simulink model "sf_slswitch_nk"  (R2020a)
settings: Solver=FixedStepAuto  StartTime=0.0  StopTime=options.T_train  FixedStep=options.dt  MaxStep=.2  RelTol=1e-3
model workspace (MAT data in the model file):
  PID_TRESH = 0.3
values from neighbouring files (symbols this model uses):
  options = trainingOptions('sgdm',      'MiniBatchSize',miniBatchSize,      'MaxEpochs',30,      'InitialLearnRate',1e-3,      'LearnRateSchedule','piecewise',      'LearnRateDropFactor',0.1,      'LearnRateDropPeriod',20,      'Shuffle','every-epoch',      'ValidationData',{XValidation,YValidation},      'ValidationFrequency',validationFrequency,      'Plots','training-progress',      'Verbose',false)    [training_lstm.m]
undefined symbols (not defined in the file or in its folder): DiscIntNeverNeededParam
libraries: neural x72, simulink x3
(part 3 of 3)

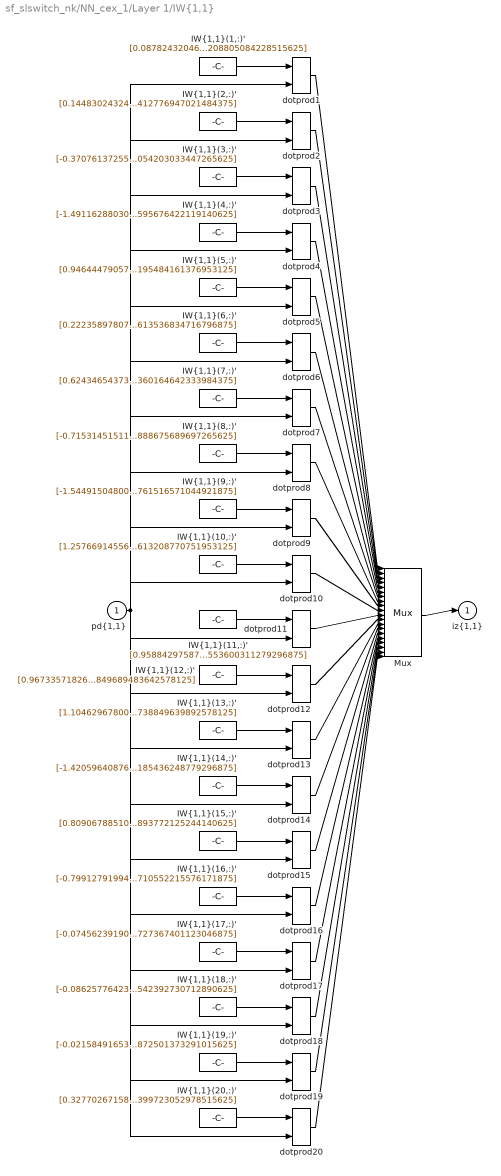
== system sf_slswitch_nk/NN_cex_1/Layer 1/IW{1,1} ==
  "pd{1,1}" : Inport  PortDimensions=6
      mask Display: e = 0.06;c1 = [120 230 180]/255;c2 = ([120 230 180]+0)/(256+128);c3 = ([120 230 180]+128)/(256+128);patch([0 1 1 0],[0 0 1 1],c1);patch([0 1 1 1-e 1-e 0+e],[0 0 1 1-e 0+e 0+e],c2);patch([0 0 1 1-e 0+e 0+e],[0 1 1 1-e 1-e 0+e],c3);plot([0 1 1 0 0],[0 0 1 1 0]);
  "IW{1,1}(1,:)'" : Constant  Value=[0.08782432046248415946632093209700542502105236053466796875;-0.78187977414949949572786636053933762013912200927734375;1.1737953327466155162284167090547271072864532470703125;1.2389070214285979876223109386046417057514190673828125;-0.721181886153456019883378758095204830169677734375;0.79676011507724897597881863475777208805084228515625]
      mask Display: e = 0.06;c1 = [120 150 230]/255;c2 = ([120 150 230]+0)/383;c3 = ([120 150 230]+128)/383;patch([0 1 1 0],[0 0 1 1],c1);patch([0 1 1 1-e 1-e 0+e],[0 0 1 1-e 0+e 0+e],c2);patch([0 0 1 1-e 0+e 0+e],[0 1 1 1-e 1-e 0+e],c3);plot([0 1 1 0 0],[0 0 1 1 0]);disp('Weights');
  "IW{1,1}(10,:)'" : Constant  Value=[1.25766914556570430505644253571517765522003173828125;-0.1306686627458673866097882410031161271035671234130859375;-0.316240354191469397182601142048952169716358184814453125;-2.075735741755533769747898986679501831531524658203125;0.478110899370217612425193465242045931518077850341796875;-0.2435194898203885405241209127780166454613208770751953125]
      mask Display: e = 0.06;c1 = [120 150 230]/255;c2 = ([120 150 230]+0)/383;c3 = ([120 150 230]+128)/383;patch([0 1 1 0],[0 0 1 1],c1);patch([0 1 1 1-e 1-e 0+e],[0 0 1 1-e 0+e 0+e],c2);patch([0 0 1 1-e 0+e 0+e],[0 1 1 1-e 1-e 0+e],c3);plot([0 1 1 0 0],[0 0 1 1 0]);disp('Weights');
  "IW{1,1}(11,:)'" : Constant  Value=[0.95884297587291189568503568807500414550304412841796875;-1.5223972203248212764492564019747078418731689453125;0.91941787050638057454676754787215031683444976806640625;0.4188723344748968013817602695780806243419647216796875;0.03411725405961420209965950789410271681845188140869140625;-1.211244817064116130467255061375908553600311279296875]
      mask Display: e = 0.06;c1 = [120 150 230]/255;c2 = ([120 150 230]+0)/383;c3 = ([120 150 230]+128)/383;patch([0 1 1 0],[0 0 1 1],c1);patch([0 1 1 1-e 1-e 0+e],[0 0 1 1-e 0+e 0+e],c2);patch([0 0 1 1-e 0+e 0+e],[0 1 1 1-e 1-e 0+e],c3);plot([0 1 1 0 0],[0 0 1 1 0]);disp('Weights');
  "IW{1,1}(12,:)'" : Constant  Value=[0.9673357182685540234245991086936555802822113037109375;-1.37966841233765524776799793471582233905792236328125;-0.0835948083749551706933544892308418639004230499267578125;-0.48948233877480706865981119335629045963287353515625;-0.59350810812291410201169128413312137126922607421875;2.1843905424894529687662725336849689483642578125]
      mask Display: e = 0.06;c1 = [120 150 230]/255;c2 = ([120 150 230]+0)/383;c3 = ([120 150 230]+128)/383;patch([0 1 1 0],[0 0 1 1],c1);patch([0 1 1 1-e 1-e 0+e],[0 0 1 1-e 0+e 0+e],c2);patch([0 0 1 1-e 0+e 0+e],[0 1 1 1-e 1-e 0+e],c3);plot([0 1 1 0 0],[0 0 1 1 0]);disp('Weights');
  "IW{1,1}(13,:)'" : Constant  Value=[1.1046296780035265161501456532278098165988922119140625;-0.1773692370934295270412661693626432679593563079833984375;1.4784971785134499722147438660613261163234710693359375;-0.92485186267143248972644187233527190983295440673828125;-1.3451227617761734034473874999093823134899139404296875;-0.60635816728712577106108483349089510738849639892578125]
      mask Display: e = 0.06;c1 = [120 150 230]/255;c2 = ([120 150 230]+0)/383;c3 = ([120 150 230]+128)/383;patch([0 1 1 0],[0 0 1 1],c1);patch([0 1 1 1-e 1-e 0+e],[0 0 1 1-e 0+e 0+e],c2);patch([0 0 1 1-e 0+e 0+e],[0 1 1 1-e 1-e 0+e],c3);plot([0 1 1 0 0],[0 0 1 1 0]);disp('Weights');
  "IW{1,1}(14,:)'" : Constant  Value=[-1.420596408769338125921422033570706844329833984375;0.038672178720716543498525652466923929750919342041015625;0.53734825594155888328629089301102794706821441650390625;0.1990017641234734513400184141573845408856868743896484375;1.0039026481054247330604312082869000732898712158203125;1.6054702518319377002598002945887856185436248779296875]
      mask Display: e = 0.06;c1 = [120 150 230]/255;c2 = ([120 150 230]+0)/383;c3 = ([120 150 230]+128)/383;patch([0 1 1 0],[0 0 1 1],c1);patch([0 1 1 1-e 1-e 0+e],[0 0 1 1-e 0+e 0+e],c2);patch([0 0 1 1-e 0+e 0+e],[0 1 1 1-e 1-e 0+e],c3);plot([0 1 1 0 0],[0 0 1 1 0]);disp('Weights');
  "IW{1,1}(15,:)'" : Constant  Value=[0.80906788510921645585227679475792683660984039306640625;-0.8477001504261389985828145654522813856601715087890625;-1.086878586388128287154586359974928200244903564453125;1.2471263492748134726895159474224783480167388916015625;-0.67997041976483962866240062794531695544719696044921875;-0.6718525676324491602287025671103037893772125244140625]
      mask Display: e = 0.06;c1 = [120 150 230]/255;c2 = ([120 150 230]+0)/383;c3 = ([120 150 230]+128)/383;patch([0 1 1 0],[0 0 1 1],c1);patch([0 1 1 1-e 1-e 0+e],[0 0 1 1-e 0+e 0+e],c2);patch([0 0 1 1-e 0+e 0+e],[0 1 1 1-e 1-e 0+e],c3);plot([0 1 1 0 0],[0 0 1 1 0]);disp('Weights');
  "IW{1,1}(16,:)'" : Constant  Value=[-0.79912791994685028473810461946413852274417877197265625;1.24789136360530772407173571991734206676483154296875;-0.45727375433479189315022495065932162106037139892578125;0.91650641770634122540428734282613731920719146728515625;-0.1754971487794872719856442699892795644700527191162109375;1.5051751167350928550803246253053657710552215576171875]
      mask Display: e = 0.06;c1 = [120 150 230]/255;c2 = ([120 150 230]+0)/383;c3 = ([120 150 230]+128)/383;patch([0 1 1 0],[0 0 1 1],c1);patch([0 1 1 1-e 1-e 0+e],[0 0 1 1-e 0+e 0+e],c2);patch([0 0 1 1-e 0+e 0+e],[0 1 1 1-e 1-e 0+e],c3);plot([0 1 1 0 0],[0 0 1 1 0]);disp('Weights');
  "IW{1,1}(17,:)'" : Constant  Value=[-0.0745623919056692952000986451821518130600452423095703125;0.51305961545316425276297422897187061607837677001953125;1.509804663729216844814118303474970161914825439453125;0.243113743854535824251428266506991349160671234130859375;1.3602358937159537699557176892994903028011322021484375;0.93869450536360143910741271611186675727367401123046875]
      mask Display: e = 0.06;c1 = [120 150 230]/255;c2 = ([120 150 230]+0)/383;c3 = ([120 150 230]+128)/383;patch([0 1 1 0],[0 0 1 1],c1);patch([0 1 1 1-e 1-e 0+e],[0 0 1 1-e 0+e 0+e],c2);patch([0 0 1 1-e 0+e 0+e],[0 1 1 1-e 1-e 0+e],c3);plot([0 1 1 0 0],[0 0 1 1 0]);disp('Weights');
  "IW{1,1}(18,:)'" : Constant  Value=[-0.08625776423674370863015070654000737704336643218994140625;-1.6481494553893709653635823997319675981998443603515625;1.3120877427964205974575406798976473510265350341796875;0.69055899618727034638965278645628131926059722900390625;0.031629039007182939424733802979972097091376781463623046875;-0.59997842039954552006975063704885542392730712890625]
      mask Display: e = 0.06;c1 = [120 150 230]/255;c2 = ([120 150 230]+0)/383;c3 = ([120 150 230]+128)/383;patch([0 1 1 0],[0 0 1 1],c1);patch([0 1 1 1-e 1-e 0+e],[0 0 1 1-e 0+e 0+e],c2);patch([0 0 1 1-e 0+e 0+e],[0 1 1 1-e 1-e 0+e],c3);plot([0 1 1 0 0],[0 0 1 1 0]);disp('Weights');
  "IW{1,1}(19,:)'" : Constant  Value=[-0.021584916530717458693633403754574828781187534332275390625;-1.4516047362781019369748491953941993415355682373046875;1.1976001156012880954904176178388297557830810546875;-0.85609977509090973146754777189926244318485260009765625;0.60165661974832840286353530245833098888397216796875;-0.77886826458716085230804537786752916872501373291015625]
      mask Display: e = 0.06;c1 = [120 150 230]/255;c2 = ([120 150 230]+0)/383;c3 = ([120 150 230]+128)/383;patch([0 1 1 0],[0 0 1 1],c1);patch([0 1 1 1-e 1-e 0+e],[0 0 1 1-e 0+e 0+e],c2);patch([0 0 1 1-e 0+e 0+e],[0 1 1 1-e 1-e 0+e],c3);plot([0 1 1 0 0],[0 0 1 1 0]);disp('Weights');
  "IW{1,1}(2,:)'" : Constant  Value=[0.1448302432457380939379021356216981075704097747802734375;1.15995447828255038302813773043453693389892578125;-1.2745630517180190910409010029979981482028961181640625;-0.1691582731432869912691074887334252707660198211669921875;-0.62289952052829578033055213381885550916194915771484375;-1.43618900402684257500141029595397412776947021484375]
      mask Display: e = 0.06;c1 = [120 150 230]/255;c2 = ([120 150 230]+0)/383;c3 = ([120 150 230]+128)/383;patch([0 1 1 0],[0 0 1 1],c1);patch([0 1 1 1-e 1-e 0+e],[0 0 1 1-e 0+e 0+e],c2);patch([0 0 1 1-e 0+e 0+e],[0 1 1 1-e 1-e 0+e],c3);plot([0 1 1 0 0],[0 0 1 1 0]);disp('Weights');
  "IW{1,1}(20,:)'" : Constant  Value=[0.327702671587350613524591835812316276133060455322265625;-0.92564673501096195185056103582610376179218292236328125;-0.6256932361109546203437048461637459695339202880859375;-1.3998360695387461749561452961643226444721221923828125;1.1316460375109504976620655725128017365932464599609375;-0.99380109900297652902878553504706360399723052978515625]
      mask Display: e = 0.06;c1 = [120 150 230]/255;c2 = ([120 150 230]+0)/383;c3 = ([120 150 230]+128)/383;patch([0 1 1 0],[0 0 1 1],c1);patch([0 1 1 1-e 1-e 0+e],[0 0 1 1-e 0+e 0+e],c2);patch([0 0 1 1-e 0+e 0+e],[0 1 1 1-e 1-e 0+e],c3);plot([0 1 1 0 0],[0 0 1 1 0]);disp('Weights');
  "IW{1,1}(3,:)'" : Constant  Value=[-0.37076137255995778030381870848941616714000701904296875;-0.1682302085218810028255376209926907904446125030517578125;0.20229206482749162443468549099634401500225067138671875;-0.966937526886006981641230595414526760578155517578125;-1.126728831267662211956803730572573840618133544921875;-1.0475569314132917586590565406368114054203033447265625]
      mask Display: e = 0.06;c1 = [120 150 230]/255;c2 = ([120 150 230]+0)/383;c3 = ([120 150 230]+128)/383;patch([0 1 1 0],[0 0 1 1],c1);patch([0 1 1 1-e 1-e 0+e],[0 0 1 1-e 0+e 0+e],c2);patch([0 0 1 1-e 0+e 0+e],[0 1 1 1-e 1-e 0+e],c3);plot([0 1 1 0 0],[0 0 1 1 0]);disp('Weights');
  "IW{1,1}(4,:)'" : Constant  Value=[-1.491162880305621829535311917425133287906646728515625;1.2351705263210615015623261569999158382415771484375;0.9765746442334293231368747001397423446178436279296875;-0.54576402531355172609295323127298615872859954833984375;0.3729944353064140738496234916965477168560028076171875;-0.63211931358371986622302074465551413595676422119140625]
      mask Display: e = 0.06;c1 = [120 150 230]/255;c2 = ([120 150 230]+0)/383;c3 = ([120 150 230]+128)/383;patch([0 1 1 0],[0 0 1 1],c1);patch([0 1 1 1-e 1-e 0+e],[0 0 1 1-e 0+e 0+e],c2);patch([0 0 1 1-e 0+e 0+e],[0 1 1 1-e 1-e 0+e],c3);plot([0 1 1 0 0],[0 0 1 1 0]);disp('Weights');
  "IW{1,1}(5,:)'" : Constant  Value=[0.94644479057617747486119696986861526966094970703125;0.213587056625421933819808373300475068390369415283203125;-1.42216624563247595602888395660556852817535400390625;-0.535583089224195507682679817662574350833892822265625;-0.87188253890788180999749101829365827143192291259765625;-0.453911766556615081658065946612623520195484161376953125]
      mask Display: e = 0.06;c1 = [120 150 230]/255;c2 = ([120 150 230]+0)/383;c3 = ([120 150 230]+128)/383;patch([0 1 1 0],[0 0 1 1],c1);patch([0 1 1 1-e 1-e 0+e],[0 0 1 1-e 0+e 0+e],c2);patch([0 0 1 1-e 0+e 0+e],[0 1 1 1-e 1-e 0+e],c3);plot([0 1 1 0 0],[0 0 1 1 0]);disp('Weights');
  "IW{1,1}(6,:)'" : Constant  Value=[0.2223589780742070143304545126738958060741424560546875;-0.99064343667998799869423010022728703916072845458984375;1.30829158201805828554142863140441477298736572265625;0.9713845979937278940496980794705450534820556640625;-0.96551633439406414627370622838498093187808990478515625;-1.246644083308769079820876868325285613536834716796875]
      mask Display: e = 0.06;c1 = [120 150 230]/255;c2 = ([120 150 230]+0)/383;c3 = ([120 150 230]+128)/383;patch([0 1 1 0],[0 0 1 1],c1);patch([0 1 1 1-e 1-e 0+e],[0 0 1 1-e 0+e 0+e],c2);patch([0 0 1 1-e 0+e 0+e],[0 1 1 1-e 1-e 0+e],c3);plot([0 1 1 0 0],[0 0 1 1 0]);disp('Weights');
  "IW{1,1}(7,:)'" : Constant  Value=[0.6243465437375361748451041421503759920597076416015625;-1.0908802446017826781599069363437592983245849609375;0.08853399815548433637868441792306839488446712493896484375;0.09527654267521283582009772317178430967032909393310546875;-1.0489358572222695631381839120876975357532501220703125;-1.160755266176609179495926582603715360164642333984375]
      mask Display: e = 0.06;c1 = [120 150 230]/255;c2 = ([120 150 230]+0)/383;c3 = ([120 150 230]+128)/383;patch([0 1 1 0],[0 0 1 1],c1);patch([0 1 1 1-e 1-e 0+e],[0 0 1 1-e 0+e 0+e],c2);patch([0 0 1 1-e 0+e 0+e],[0 1 1 1-e 1-e 0+e],c3);plot([0 1 1 0 0],[0 0 1 1 0]);disp('Weights');
  "IW{1,1}(8,:)'" : Constant  Value=[-0.71531451511786270369697149362764321267604827880859375;1.0810010007743124926804512142552994191646575927734375;0.909604153527625580721860387711785733699798583984375;-0.5533589940715819555094867610023356974124908447265625;0.26850883021074001266725872483220882713794708251953125;-1.4328804786490911826746241786167956888675689697265625]
      mask Display: e = 0.06;c1 = [120 150 230]/255;c2 = ([120 150 230]+0)/383;c3 = ([120 150 230]+128)/383;patch([0 1 1 0],[0 0 1 1],c1);patch([0 1 1 1-e 1-e 0+e],[0 0 1 1-e 0+e 0+e],c2);patch([0 0 1 1-e 0+e 0+e],[0 1 1 1-e 1-e 0+e],c3);plot([0 1 1 0 0],[0 0 1 1 0]);disp('Weights');
  "IW{1,1}(9,:)'" : Constant  Value=[-1.54491504800237411387797692441381514072418212890625;-0.87105103692524188385704064785386435687541961669921875;0.11190116102801002384570239200911601074039936065673828125;-0.073196360579186714456767504088929854333400726318359375;0.2625267794875891791406274933251552283763885498046875;2.117987303839647506009669086779467761516571044921875]
      mask Display: e = 0.06;c1 = [120 150 230]/255;c2 = ([120 150 230]+0)/383;c3 = ([120 150 230]+128)/383;patch([0 1 1 0],[0 0 1 1],c1);patch([0 1 1 1-e 1-e 0+e],[0 0 1 1-e 0+e 0+e],c2);patch([0 0 1 1-e 0+e 0+e],[0 1 1 1-e 1-e 0+e],c3);plot([0 1 1 0 0],[0 0 1 1 0]);disp('Weights');
  Mux : Mux  Inputs=20
      mask Display: e = 0.06;c1 = [120 150 230]/255;c2 = ([120 150 230]+0)/383;c3 = ([120 150 230]+128)/383;patch([0 1 1 0],[0 0 1 1],c1);patch([0 1 1 1-e 1-e 0+e],[0 0 1 1-e 0+e 0+e],c2);patch([0 0 1 1-e 0+e 0+e],[0 1 1 1-e 1-e 0+e],c3);plot([0 1 1 0 0],[0 0 1 1 0]);disp('Mux');
  dotprod{1..20} (20 alike) : neural/Weight Functions/dotprod
  "iz{1,1}" : Outport
      mask Display: e = 0.06;c1 = [120 230 180]/255;c2 = ([120 230 180]+0)/(256+128);c3 = ([120 230 180]+128)/(256+128);patch([0 1 1 0],[0 0 1 1],c1);patch([0 1 1 1-e 1-e 0+e],[0 0 1 1-e 0+e 0+e],c2);patch([0 0 1 1-e 0+e 0+e],[0 1 1 1-e 1-e 0+e],c3);plot([0 1 1 0 0],[0 0 1 1 0]);
  wires:
  "IW{1,1}(1,:)'"/1 -> dotprod1/1
  "pd{1,1}"/1 -> dotprod1/2, dotprod2/2, dotprod3/2, dotprod4/2, dotprod5/2, dotprod6/2, dotprod7/2, dotprod8/2, dotprod9/2, dotprod10/2, dotprod11/2, dotprod12/2, dotprod13/2, dotprod14/2, dotprod15/2, dotprod16/2, dotprod17/2, dotprod18/2, dotprod19/2, dotprod20/2
  dotprod1/1 -> Mux/1
  "IW{1,1}(2,:)'"/1 -> dotprod2/1
  dotprod2/1 -> Mux/2
  "IW{1,1}(3,:)'"/1 -> dotprod3/1
  dotprod3/1 -> Mux/3
  "IW{1,1}(4,:)'"/1 -> dotprod4/1
  dotprod4/1 -> Mux/4
  "IW{1,1}(5,:)'"/1 -> dotprod5/1
  dotprod5/1 -> Mux/5
  "IW{1,1}(6,:)'"/1 -> dotprod6/1
  dotprod6/1 -> Mux/6
  "IW{1,1}(7,:)'"/1 -> dotprod7/1
  dotprod7/1 -> Mux/7
  "IW{1,1}(8,:)'"/1 -> dotprod8/1
  dotprod8/1 -> Mux/8
  "IW{1,1}(9,:)'"/1 -> dotprod9/1
  dotprod9/1 -> Mux/9
  "IW{1,1}(10,:)'"/1 -> dotprod10/1
  dotprod10/1 -> Mux/10
  "IW{1,1}(11,:)'"/1 -> dotprod11/1
  dotprod11/1 -> Mux/11
  "IW{1,1}(12,:)'"/1 -> dotprod12/1
  dotprod12/1 -> Mux/12
  "IW{1,1}(13,:)'"/1 -> dotprod13/1
  dotprod13/1 -> Mux/13
  "IW{1,1}(14,:)'"/1 -> dotprod14/1
  dotprod14/1 -> Mux/14
  "IW{1,1}(15,:)'"/1 -> dotprod15/1
  dotprod15/1 -> Mux/15
  "IW{1,1}(16,:)'"/1 -> dotprod16/1
  dotprod16/1 -> Mux/16
  "IW{1,1}(17,:)'"/1 -> dotprod17/1
  dotprod17/1 -> Mux/17
  "IW{1,1}(18,:)'"/1 -> dotprod18/1
  dotprod18/1 -> Mux/18
  "IW{1,1}(19,:)'"/1 -> dotprod19/1
  dotprod19/1 -> Mux/19
  "IW{1,1}(20,:)'"/1 -> dotprod20/1
  dotprod20/1 -> Mux/20
  Mux/1 -> "iz{1,1}"/1

== system sf_slswitch_nk/NN_cex_1/Layer 2/Delays 1 ==
  "p{2}" : Inport  PortDimensions=20
      mask Display: e = 0.06;c1 = [120 230 180]/255;c2 = ([120 230 180]+0)/(256+128);c3 = ([120 230 180]+128)/(256+128);patch([0 1 1 0],[0 0 1 1],c1);patch([0 1 1 1-e 1-e 0+e],[0 0 1 1-e 0+e 0+e],c2);patch([0 0 1 1-e 0+e 0+e],[0 1 1 1-e 1-e 0+e],c3);plot([0 1 1 0 0],[0 0 1 1 0]);
  mux : Mux  Inputs=1
      mask Display: e = 0.06;c1 = [120 150 230]/255;c2 = ([120 150 230]+0)/383;c3 = ([120 150 230]+128)/383;patch([0 1 1 0],[0 0 1 1],c1);patch([0 1 1 1-e 1-e 0+e],[0 0 1 1-e 0+e 0+e],c2);patch([0 0 1 1-e 0+e 0+e],[0 1 1 1-e 1-e 0+e],c3);plot([0 1 1 0 0],[0 0 1 1 0]);disp('Mux')
  "pd{2,1}" : Outport
      mask Display: e = 0.06;c1 = [120 230 180]/255;c2 = ([120 230 180]+0)/(256+128);c3 = ([120 230 180]+128)/(256+128);patch([0 1 1 0],[0 0 1 1],c1);patch([0 1 1 1-e 1-e 0+e],[0 0 1 1-e 0+e 0+e],c2);patch([0 0 1 1-e 0+e 0+e],[0 1 1 1-e 1-e 0+e],c3);plot([0 1 1 0 0],[0 0 1 1 0]);
  wires:
  "p{2}"/1 -> mux/1
  mux/1 -> "pd{2,1}"/1

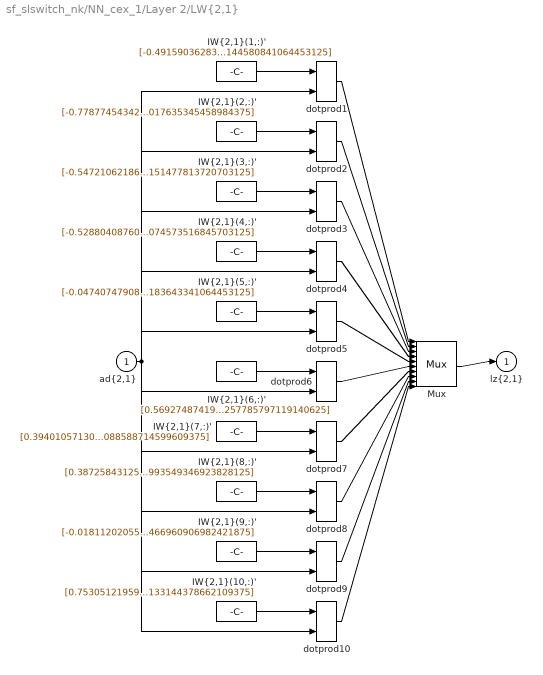
== system sf_slswitch_nk/NN_cex_1/Layer 2/LW{2,1} ==
  "ad{2,1}" : Inport  PortDimensions=20
      mask Display: e = 0.06;c1 = [120 230 180]/255;c2 = ([120 230 180]+0)/(256+128);c3 = ([120 230 180]+128)/(256+128);patch([0 1 1 0],[0 0 1 1],c1);patch([0 1 1 1-e 1-e 0+e],[0 0 1 1-e 0+e 0+e],c2);patch([0 0 1 1-e 0+e 0+e],[0 1 1 1-e 1-e 0+e],c3);plot([0 1 1 0 0],[0 0 1 1 0]);
  "IW{2,1}(1,:)'" : Constant  Value=[-0.491590362838410843693282004096545279026031494140625;0.09153558772017998668157900965525186620652675628662109375;0.53913620049723587346335307302069850265979766845703125;0.28986214268498233792570317746140062808990478515625;-0.098872454446192914456759126551332883536815643310546875;-0.187324447372830882319050260775838978588581085205078125;0.236253529461758871033083551083109341561794281005859375;0.5875443481423918701267439246294088661670684814453125;0.2365904294687373177197287077433429658412933349609375;-0.36194560670800945967329198538209311664104461669921875;-0.5079024928489610513082652687444351613521575927734375;-0.372571443628679777049228505347855389118194580078125;0.12093583417952176450871348833970841951668262481689453125;-0.362502777161662292915167427054257132112979888916015625;0.50843366259362554604450679107685573399066925048828125;-0.41560452030535655065790479056886397302150726318359375;0.256861168211626689217297325740219093859195709228515625;-0.2213914820522025761473372540422133170068264007568359375;0.037440396125606560662202326739134150557219982147216796875;0.457230844134753955376737621918437071144580841064453125]
      mask Display: e = 0.06;c1 = [120 150 230]/255;c2 = ([120 150 230]+0)/383;c3 = ([120 150 230]+128)/383;patch([0 1 1 0],[0 0 1 1],c1);patch([0 1 1 1-e 1-e 0+e],[0 0 1 1-e 0+e 0+e],c2);patch([0 0 1 1-e 0+e 0+e],[0 1 1 1-e 1-e 0+e],c3);plot([0 1 1 0 0],[0 0 1 1 0]);disp('weights');
  "IW{2,1}(10,:)'" : Constant  Value=[0.75305121959948040366583654758869670331478118896484375;-0.3260684130024174010031856596469879150390625;-0.374803912786967174941565872359205968677997589111328125;-0.42045135255658883099982858766452409327030181884765625;0.393471966963337582701143446684000082314014434814453125;0.375054346973890229133274942796560935676097869873046875;0.2989752325221666229282391213928349316120147705078125;-0.688885140013455465890501727699302136898040771484375;0.358758212849716706660530007866327650845050811767578125;-0.8248494367770897728320278474711813032627105712890625;0.60260676331586726650613172751036472618579864501953125;-0.73445901643811561942953858306282199919223785400390625;0.2205739585100955080232409954987815581262111663818359375;0.71227553523238673616191363180405460298061370849609375;0.6516926017157469441798411935451440513134002685546875;0.2726156313484942028679824943537823855876922607421875;-0.3069395915147554720903144698240794241428375244140625;0.54386527491213143559178888608585111796855926513671875;-0.160428031831243822491472883484675548970699310302734375;0.194338689113902451932602843953645788133144378662109375]
      mask Display: e = 0.06;c1 = [120 150 230]/255;c2 = ([120 150 230]+0)/383;c3 = ([120 150 230]+128)/383;patch([0 1 1 0],[0 0 1 1],c1);patch([0 1 1 1-e 1-e 0+e],[0 0 1 1-e 0+e 0+e],c2);patch([0 0 1 1-e 0+e 0+e],[0 1 1 1-e 1-e 0+e],c3);plot([0 1 1 0 0],[0 0 1 1 0]);disp('weights');
  "IW{2,1}(2,:)'" : Constant  Value=[-0.77877454342913432494555081575526855885982513427734375;0.441383032730336022364525661032530479133129119873046875;-0.251052647469331369212142135438625700771808624267578125;0.01653276142955795169342536610201932489871978759765625;-0.59984645072742959204248336391174234449863433837890625;0.74448563957262481327603609315701760351657867431640625;-0.163011531951689381259029687498696148395538330078125;0.1637861574392550367829102242467342875897884368896484375;-0.10147583382602155810392474677428253926336765289306640625;0.6199959878969651949631725074141286313533782958984375;-0.556560585377592786926470580510795116424560546875;0.77146041768374551406139971732045523822307586669921875;-0.2051901400079843840185134240527986548840999603271484375;-0.0192216131581010307716184115633950568735599517822265625;0.86674916935437185117052649729885160923004150390625;0.269559052351910743983154361558263190090656280517578125;0.2454882084512731432734966574571444652974605560302734375;0.324690879650742780793137853834195993840694427490234375;0.250330019953576898839031628085649572312831878662109375;-0.3491341460419279396631964118569158017635345458984375]
      mask Display: e = 0.06;c1 = [120 150 230]/255;c2 = ([120 150 230]+0)/383;c3 = ([120 150 230]+128)/383;patch([0 1 1 0],[0 0 1 1],c1);patch([0 1 1 1-e 1-e 0+e],[0 0 1 1-e 0+e 0+e],c2);patch([0 0 1 1-e 0+e 0+e],[0 1 1 1-e 1-e 0+e],c3);plot([0 1 1 0 0],[0 0 1 1 0]);disp('weights');
  "IW{2,1}(3,:)'" : Constant  Value=[-0.54721062186453994780066523162531666457653045654296875;0.35963325219462716209051222904236055910587310791015625;0.310171878633505648803492249498958699405193328857421875;-0.355214818614143890140866233195993117988109588623046875;-0.35826823774047855675206619707751087844371795654296875;0.59190758871869508794816283625550568103790283203125;0.244587132338854207347367264446802437305450439453125;0.676231222299827461341692469432018697261810302734375;0.334998849685998578706858097575604915618896484375;-0.3927938690434251700622780845151282846927642822265625;0.59523218778234754378075876957154832780361175537109375;-0.26782939241242764705219769894029013812541961669921875;-0.12149629693078932424210591989321983419358730316162109375;-0.5781848855833555678174207059782929718494415283203125;-0.321982299760499357521581487162620760500431060791015625;-0.2085323873828421603615623780569876544177532196044921875;0.558010739506813902011117534129880368709564208984375;0.44381755439858705525324467089376412332057952880859375;0.1734132742370666502296217004186473786830902099609375;-0.6048978397542523754992771500837989151477813720703125]
      mask Display: e = 0.06;c1 = [120 150 230]/255;c2 = ([120 150 230]+0)/383;c3 = ([120 150 230]+128)/383;patch([0 1 1 0],[0 0 1 1],c1);patch([0 1 1 1-e 1-e 0+e],[0 0 1 1-e 0+e 0+e],c2);patch([0 0 1 1-e 0+e 0+e],[0 1 1 1-e 1-e 0+e],c3);plot([0 1 1 0 0],[0 0 1 1 0]);disp('weights');
  "IW{2,1}(4,:)'" : Constant  Value=[-0.5288040876066730788807035423815250396728515625;-0.12058629158413725068754729363718070089817047119140625;0.287618107827734059700475199861102737486362457275390625;-0.11025708650445709135823335600434802472591400146484375;0.175148355500430563669311823105090297758579254150390625;0.17248802275310470832891951431520283222198486328125;-0.431099714626743402146047401402029208838939666748046875;-0.386386624067918182934278092943714000284671783447265625;0.478441160453836389354620450831134803593158721923828125;0.2288021055062318398487519743866869248449802398681640625;-0.274526400229313960466015487327240407466888427734375;0.56342733208960626978267782760667614638805389404296875;-0.300978459968216094377879699095501564443111419677734375;0.437178179335386551951359024315024726092815399169921875;-0.05734225737338206896342995833038003183901309967041015625;0.181127732497251725529707755413255654275417327880859375;-0.382609890761644866330470904358662664890289306640625;0.28013200624474243749517654578085057437419891357421875;0.519547545879515570987905448419041931629180908203125;0.63049438096737386860723972858977504074573516845703125]
      mask Display: e = 0.06;c1 = [120 150 230]/255;c2 = ([120 150 230]+0)/383;c3 = ([120 150 230]+128)/383;patch([0 1 1 0],[0 0 1 1],c1);patch([0 1 1 1-e 1-e 0+e],[0 0 1 1-e 0+e 0+e],c2);patch([0 0 1 1-e 0+e 0+e],[0 1 1 1-e 1-e 0+e],c3);plot([0 1 1 0 0],[0 0 1 1 0]);disp('weights');
  "IW{2,1}(5,:)'" : Constant  Value=[-0.047407479086184055316888219522297731600701808929443359375;0.6817124416683757459622938768006861209869384765625;0.15898075041414283514740191094460897147655487060546875;-0.23570292887630650557895251040463335812091827392578125;-0.57616431494863562523534028514404781162738800048828125;0.97740595933983553944557343129417859017848968505859375;-0.035424998297084002440993089066978427581489086151123046875;0.8429529431915916415363199121202342212200164794921875;-0.92952130083627071410745656976359896361827850341796875;-0.1650025805505259401950723940899479202926158905029296875;0.0458112662697143513401698555753682740032672882080078125;-0.51472079611698073886572046831133775413036346435546875;-0.2147134890184759503650724354884005151689052581787109375;0.3009307468411994701540379537618719041347503662109375;-0.50902089304013375947732811255264095962047576904296875;0.0714043768121936095472079841783852316439151763916015625;-0.48823829383933115000360203339369036257266998291015625;0.3651420006460466272102394214016385376453399658203125;-0.163209777690640767122687293522176332771778106689453125;-0.2198929880588023355603155550852534361183643341064453125]
      mask Display: e = 0.06;c1 = [120 150 230]/255;c2 = ([120 150 230]+0)/383;c3 = ([120 150 230]+128)/383;patch([0 1 1 0],[0 0 1 1],c1);patch([0 1 1 1-e 1-e 0+e],[0 0 1 1-e 0+e 0+e],c2);patch([0 0 1 1-e 0+e 0+e],[0 1 1 1-e 1-e 0+e],c3);plot([0 1 1 0 0],[0 0 1 1 0]);disp('weights');
  "IW{2,1}(6,:)'" : Constant  Value=[0.56927487419209132912811810456332750618457794189453125;0.0964248338569875518277996206961688585579395294189453125;0.53068784843067395851079481872147880494594573974609375;-0.41879976656768491682925059649278409779071807861328125;-0.132000833034666531506928777162102051079273223876953125;0.188733076523335208118936634491547010838985443115234375;-0.437083852659319649358593551369267515838146209716796875;-0.3212725201176052092222334977122955024242401123046875;-0.376298123159041486562870204579667188227176666259765625;-0.37253083537160802674037540782592259347438812255859375;-0.00089507108511371609275986127585156282293610274791717529296875;0.48208847549187705538997761323116719722747802734375;0.256839521638566103955980679529602639377117156982421875;0.314408237479162522287623460215399973094463348388671875;0.40417843844262579811044133748509921133518218994140625;-0.0253262404009013918082526828357003978453576564788818359375;0.313632017884898584014763400773517787456512451171875;0.54634428165702575430628940011956728994846343994140625;-0.0157081414607670270811023982560072909109294414520263671875;0.03174977849280914699026112657520570792257785797119140625]
      mask Display: e = 0.06;c1 = [120 150 230]/255;c2 = ([120 150 230]+0)/383;c3 = ([120 150 230]+128)/383;patch([0 1 1 0],[0 0 1 1],c1);patch([0 1 1 1-e 1-e 0+e],[0 0 1 1-e 0+e 0+e],c2);patch([0 0 1 1-e 0+e 0+e],[0 1 1 1-e 1-e 0+e],c3);plot([0 1 1 0 0],[0 0 1 1 0]);disp('weights');
  "IW{2,1}(7,:)'" : Constant  Value=[0.3940105713042798551981604759930633008480072021484375;-0.1738459504246700759733101904203067533671855926513671875;0.27901220074907995272184280111105181276798248291015625;-0.5063197207027572144255600505857728421688079833984375;0.38598654481844019148439883792889304459095001220703125;-0.344247002528806300691854858087026514112949371337890625;0.08233134008832214412176853102209861390292644500732421875;-0.1406199280171001320116630495249410159885883331298828125;-0.483698766782882094705797726419405080378055572509765625;0.38266394217537491595493293061736039817333221435546875;-1.0985645521483677899965414326288737356662750244140625;0.84912234342618286841997132796677760779857635498046875;-0.0603943569737682428577585369566804729402065277099609375;0.5285984337608160554822234189487062394618988037109375;-0.0022227474997935613154620426712426706217229366302490234375;0.6067215383125541539044434102834202349185943603515625;-0.331845109066125354413401282727136276662349700927734375;0.409371532238706203887801393648260273039340972900390625;0.33678512418631634250942852304433472454547882080078125;0.435096675695478329881638046572334133088588714599609375]
      mask Display: e = 0.06;c1 = [120 150 230]/255;c2 = ([120 150 230]+0)/383;c3 = ([120 150 230]+128)/383;patch([0 1 1 0],[0 0 1 1],c1);patch([0 1 1 1-e 1-e 0+e],[0 0 1 1-e 0+e 0+e],c2);patch([0 0 1 1-e 0+e 0+e],[0 1 1 1-e 1-e 0+e],c3);plot([0 1 1 0 0],[0 0 1 1 0]);disp('weights');
  "IW{2,1}(8,:)'" : Constant  Value=[0.387258431253234169933108432815060950815677642822265625;0.2961032210837466482900026676361449062824249267578125;0.36557177655976091923406556816189549863338470458984375;0.3959118086086161891756773911765776574611663818359375;0.72607123155116559676258702893392182886600494384765625;-0.475669568537124776153035554671077989041805267333984375;-0.260490351238776340903058326148311607539653778076171875;-0.057587141567412271359049924512873985804617404937744140625;-0.353253584571080969656264869627193547785282135009765625;0.61249358289222755047376267611980438232421875;0.13725992262079333983137985342182219028472900390625;0.06318261054722727754207056705126888118684291839599609375;0.5528030330867566011221470034797675907611846923828125;0.5800628529446327785734638382564298808574676513671875;0.278304396984638435785797128119156695902347564697265625;0.72861502699942992666848340377327986061573028564453125;0.33649053036731768617784155139815993607044219970703125;-0.1319690903451178620731099044860457070171833038330078125;-0.1783999502583830942814557829478872008621692657470703125;-0.324409377570461732176454461296088993549346923828125]
      mask Display: e = 0.06;c1 = [120 150 230]/255;c2 = ([120 150 230]+0)/383;c3 = ([120 150 230]+128)/383;patch([0 1 1 0],[0 0 1 1],c1);patch([0 1 1 1-e 1-e 0+e],[0 0 1 1-e 0+e 0+e],c2);patch([0 0 1 1-e 0+e 0+e],[0 1 1 1-e 1-e 0+e],c3);plot([0 1 1 0 0],[0 0 1 1 0]);disp('weights');
  "IW{2,1}(9,:)'" : Constant  Value=[-0.018112020559307169531582104582412284798920154571533203125;-0.2479362254143927246641254669157206080853939056396484375;-0.281293634999924158091033632445032708346843719482421875;0.53376970667455780894528061253367923200130462646484375;-0.62081621983989332402842364899697713553905487060546875;0.00254759436079938540731237850422985502518713474273681640625;-0.0959419444015851274887296540327952243387699127197265625;-0.26005572483561512076022381734219379723072052001953125;0.47366112132426663183792925337911583483219146728515625;-0.2465795616014130053894604088782216422259807586669921875;-0.420365486658341558356966061182902194559574127197265625;0.61394968969644103662375300700659863650798797607421875;0.2998525051883620395898333299555815756320953369140625;0.27427334066912389953785122997942380607128143310546875;-0.61379471947160768596774005345650948584079742431640625;0.2946315797099281486026711718295700848102569580078125;0.52213052862831654810094050844782032072544097900390625;0.63632591996082421559322028770111501216888427734375;-0.0034006561171643239806228198318649447173811495304107666015625;0.447588888253873384837078219788963906466960906982421875]
      mask Display: e = 0.06;c1 = [120 150 230]/255;c2 = ([120 150 230]+0)/383;c3 = ([120 150 230]+128)/383;patch([0 1 1 0],[0 0 1 1],c1);patch([0 1 1 1-e 1-e 0+e],[0 0 1 1-e 0+e 0+e],c2);patch([0 0 1 1-e 0+e 0+e],[0 1 1 1-e 1-e 0+e],c3);plot([0 1 1 0 0],[0 0 1 1 0]);disp('weights');
  Mux : Mux  Inputs=10
      mask Display: e = 0.06;c1 = [120 150 230]/255;c2 = ([120 150 230]+0)/383;c3 = ([120 150 230]+128)/383;patch([0 1 1 0],[0 0 1 1],c1);patch([0 1 1 1-e 1-e 0+e],[0 0 1 1-e 0+e 0+e],c2);patch([0 0 1 1-e 0+e 0+e],[0 1 1 1-e 1-e 0+e],c3);plot([0 1 1 0 0],[0 0 1 1 0]);disp('Mux');
  dotprod{1..10} (10 alike) : neural/Weight Functions/dotprod
  "lz{2,1}" : Outport
      mask Display: e = 0.06;c1 = [120 230 180]/255;c2 = ([120 230 180]+0)/(256+128);c3 = ([120 230 180]+128)/(256+128);patch([0 1 1 0],[0 0 1 1],c1);patch([0 1 1 1-e 1-e 0+e],[0 0 1 1-e 0+e 0+e],c2);patch([0 0 1 1-e 0+e 0+e],[0 1 1 1-e 1-e 0+e],c3);plot([0 1 1 0 0],[0 0 1 1 0]);
  wires:
  "IW{2,1}(1,:)'"/1 -> dotprod1/1
  "ad{2,1}"/1 -> dotprod1/2, dotprod2/2, dotprod3/2, dotprod4/2, dotprod5/2, dotprod6/2, dotprod7/2, dotprod8/2, dotprod9/2, dotprod10/2
  dotprod1/1 -> Mux/1
  "IW{2,1}(2,:)'"/1 -> dotprod2/1
  dotprod2/1 -> Mux/2
  "IW{2,1}(3,:)'"/1 -> dotprod3/1
  dotprod3/1 -> Mux/3
  "IW{2,1}(4,:)'"/1 -> dotprod4/1
  dotprod4/1 -> Mux/4
  "IW{2,1}(5,:)'"/1 -> dotprod5/1
  dotprod5/1 -> Mux/5
  "IW{2,1}(6,:)'"/1 -> dotprod6/1
  dotprod6/1 -> Mux/6
  "IW{2,1}(7,:)'"/1 -> dotprod7/1
  dotprod7/1 -> Mux/7
  "IW{2,1}(8,:)'"/1 -> dotprod8/1
  dotprod8/1 -> Mux/8
  "IW{2,1}(9,:)'"/1 -> dotprod9/1
  dotprod9/1 -> Mux/9
  "IW{2,1}(10,:)'"/1 -> dotprod10/1
  dotprod10/1 -> Mux/10
  Mux/1 -> "lz{2,1}"/1

== system sf_slswitch_nk/NN_cex_1/Layer 3/Delays 1 ==
  "p{3}" : Inport  PortDimensions=10
      mask Display: e = 0.06;c1 = [120 230 180]/255;c2 = ([120 230 180]+0)/(256+128);c3 = ([120 230 180]+128)/(256+128);patch([0 1 1 0],[0 0 1 1],c1);patch([0 1 1 1-e 1-e 0+e],[0 0 1 1-e 0+e 0+e],c2);patch([0 0 1 1-e 0+e 0+e],[0 1 1 1-e 1-e 0+e],c3);plot([0 1 1 0 0],[0 0 1 1 0]);
  mux : Mux  Inputs=1
      mask Display: e = 0.06;c1 = [120 150 230]/255;c2 = ([120 150 230]+0)/383;c3 = ([120 150 230]+128)/383;patch([0 1 1 0],[0 0 1 1],c1);patch([0 1 1 1-e 1-e 0+e],[0 0 1 1-e 0+e 0+e],c2);patch([0 0 1 1-e 0+e 0+e],[0 1 1 1-e 1-e 0+e],c3);plot([0 1 1 0 0],[0 0 1 1 0]);disp('Mux')
  "pd{3,2}" : Outport
      mask Display: e = 0.06;c1 = [120 230 180]/255;c2 = ([120 230 180]+0)/(256+128);c3 = ([120 230 180]+128)/(256+128);patch([0 1 1 0],[0 0 1 1],c1);patch([0 1 1 1-e 1-e 0+e],[0 0 1 1-e 0+e 0+e],c2);patch([0 0 1 1-e 0+e 0+e],[0 1 1 1-e 1-e 0+e],c3);plot([0 1 1 0 0],[0 0 1 1 0]);
  wires:
  "p{3}"/1 -> mux/1
  mux/1 -> "pd{3,2}"/1

== system sf_slswitch_nk/NN_cex_1/Layer 3/LW{3,2} ==
  "ad{3,2}" : Inport  PortDimensions=10
      mask Display: e = 0.06;c1 = [120 230 180]/255;c2 = ([120 230 180]+0)/(256+128);c3 = ([120 230 180]+128)/(256+128);patch([0 1 1 0],[0 0 1 1],c1);patch([0 1 1 1-e 1-e 0+e],[0 0 1 1-e 0+e 0+e],c2);patch([0 0 1 1-e 0+e 0+e],[0 1 1 1-e 1-e 0+e],c3);plot([0 1 1 0 0],[0 0 1 1 0]);
  "IW{3,2}(1,:)'" : Constant  Value=[-0.0763051436986283970753675021114759147167205810546875;-1.2751206298841035735591731281601823866367340087890625;-0.9314503721775029276841451064683496952056884765625;-0.8943677153502556098629838743363507091999053955078125;-1.068478159183759768069421625114046037197113037109375;0.017334965141479134753677016078654560260474681854248046875;-1.3056916227918833328658365644514560699462890625;0.94753297375811207370333022481645457446575164794921875;-0.4254536794848673419977558296523056924343109130859375;1.15709984208541438732709139003418385982513427734375]
      mask Display: e = 0.06;c1 = [120 150 230]/255;c2 = ([120 150 230]+0)/383;c3 = ([120 150 230]+128)/383;patch([0 1 1 0],[0 0 1 1],c1);patch([0 1 1 1-e 1-e 0+e],[0 0 1 1-e 0+e 0+e],c2);patch([0 0 1 1-e 0+e 0+e],[0 1 1 1-e 1-e 0+e],c3);plot([0 1 1 0 0],[0 0 1 1 0]);disp('weights');
  Mux : Mux  Inputs=1
      mask Display: e = 0.06;c1 = [120 150 230]/255;c2 = ([120 150 230]+0)/383;c3 = ([120 150 230]+128)/383;patch([0 1 1 0],[0 0 1 1],c1);patch([0 1 1 1-e 1-e 0+e],[0 0 1 1-e 0+e 0+e],c2);patch([0 0 1 1-e 0+e 0+e],[0 1 1 1-e 1-e 0+e],c3);plot([0 1 1 0 0],[0 0 1 1 0]);disp('Mux');
  dotprod1 : neural/Weight Functions/dotprod
  "lz{3,2}" : Outport
      mask Display: e = 0.06;c1 = [120 230 180]/255;c2 = ([120 230 180]+0)/(256+128);c3 = ([120 230 180]+128)/(256+128);patch([0 1 1 0],[0 0 1 1],c1);patch([0 1 1 1-e 1-e 0+e],[0 0 1 1-e 0+e 0+e],c2);patch([0 0 1 1-e 0+e 0+e],[0 1 1 1-e 1-e 0+e],c3);plot([0 1 1 0 0],[0 0 1 1 0]);
  wires:
  "IW{3,2}(1,:)'"/1 -> dotprod1/1
  "ad{3,2}"/1 -> dotprod1/2
  dotprod1/1 -> Mux/1
  Mux/1 -> "lz{3,2}"/1

== stateflow chart sf_slswitch_nk/SwitchingController ==
  state STEADY
    entry: u = 0;
  state P
    du:
    u = p_control(e);
    state u = p_control(e) [function]
  state PID
    du:
    u = pid_control(e);
    state u = pid_control(e) [function]
  (default) -> STEADY
  STEADY -> P : [e > 0.01]
  P -> PID : [e < PID_TRESH]
  data: e function_input; u function_output; e function_input; u function_output; e input; u output double; PID output boolean; PID_TRESH parameter; P output boolean
